simulink model "sfcndemo_matadd"  (Simulink 7.6)
settings: Solver=FixedStepDiscrete  StartTime=0.0  StopTime=10.0  RelTol=1e-3
Description:
  | Matrix-Add (Bias) Using One Input and One Parameter C-MEX S-function
settings Model: Creator=The MathWorks Inc.  ExtModeAutoUpdateStatusClock=off
settings DataIOCC: SaveOutput=off  OutputSaveName=y1,y2,y3,y4
settings OptimizationCC: BlockReduction=off  BooleanDataType=off  InlineInvariantSignals=on  InitFltsAndDblsToZero=on
settings DebuggingCC: SaveWithParameterizedLinksMsg=none  SignalResolutionControl=TryResolveAllWithWarning  SolverPrmCheckMsg=none  MultiTaskDSMMsg=warning  MultiTaskCondExecSysMsg=none
settings HardwareCC: TargetUnknown=on
settings RTWCC: IncludeERTFirstTime=on
settings CodeAppCC: CustomSymbolStrFcn=$F$N$M
settings GRTTargetCC: TargetFcnLib=ansi_tfl_tmw.mat

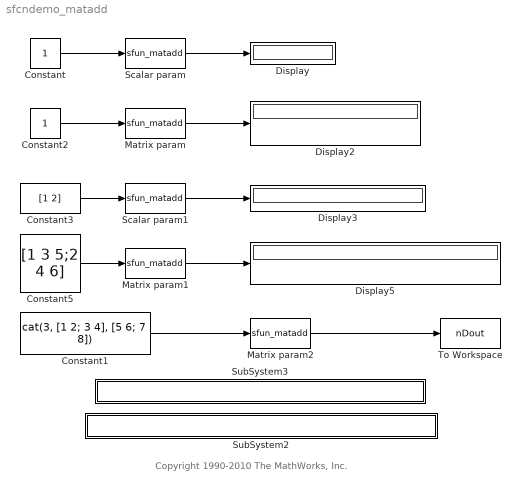
== system sfcndemo_matadd ==
  note: Copyright 1990-2010 The MathWorks, Inc.
  Constant : Constant  VectorParams1D=off
  Constant1 : Constant  Value=cat(3, [1 2; 3 4], [5 6; 7 8])  VectorParams1D=off
  Constant2 : Constant  VectorParams1D=off
  Constant3 : Constant  Value=[1 2]  VectorParams1D=off
  Constant5 : Constant  Value=[1 3 5;2 4 6]  VectorParams1D=off
  Display{,2..3,5} (4 alike) : Display
  Matrix param : S-Function  FunctionName=sfun_matadd  Parameters=Operand  EnableBusSupport=off  mask(Matrix add){Operand=[1 3; 2 4]}
      mask prompts: Operand "Operand 1:"
      settings: AttributesFormatString=Param = %<Operand>
      mask Display: disp('Matrix\n Add ')
  Matrix param1 : S-Function  FunctionName=sfun_matadd  Parameters=Operand  EnableBusSupport=off  mask(Matrix add){Operand=[1 3 5;2 4 6]}
      mask prompts: Operand "Operand 1:"
      settings: AttributesFormatString=Param = %<Operand>
      mask Display: disp('Matrix\n Add ')
  Matrix param2 : S-Function  FunctionName=sfun_matadd  Parameters=Operand  EnableBusSupport=off  mask(Matrix add){Operand=cat(3, [1 2; 3 4], [5 6; 7 8])}
      mask prompts: Operand "Operand 1:"
      settings: AttributesFormatString=Param = %<Operand>
      mask Display: disp('Matrix\n Add ')
  Scalar param : S-Function  FunctionName=sfun_matadd  Parameters=Operand  EnableBusSupport=off  mask(Matrix add){Operand=1}
      mask prompts: Operand "Operand 1:"
      settings: AttributesFormatString=Param = %<Operand>
      mask Display: disp('Matrix\n Add ')
  Scalar param1 : S-Function  FunctionName=sfun_matadd  Parameters=Operand  EnableBusSupport=off  mask(Matrix add){Operand=1}
      mask prompts: Operand "Operand 1:"
      settings: AttributesFormatString=Param = %<Operand>
      mask Display: disp('Matrix\n Add ')
  SubSystem2 : Subsystem  mask{filename=sfun_matadd.tlc}
      mask init:
      | x=sfundemo_maskdisp;
      settings: AttributesFormatString=\n  OpenFcn=sfundemo_openfcn
      mask Display: disp(x);
  SubSystem3 : Subsystem  mask{filename=sfun_matadd.c}
      mask init:
      | x=sfundemo_maskdisp;
      settings: AttributesFormatString=\n  OpenFcn=sfundemo_openfcn
      mask Display: disp(x);
  To Workspace : ToWorkspace  VariableName=nDout  SampleTime=-1  SaveFormat=Structure
  wires:
  Constant/1 -> Scalar param/1
  Scalar param/1 -> Display/1
  Constant2/1 -> Matrix param/1
  Matrix param/1 -> Display2/1
  Constant3/1 -> Scalar param1/1
  Scalar param1/1 -> Display3/1
  Constant5/1 -> Matrix param1/1
  Matrix param1/1 -> Display5/1
  Constant1/1 -> Matrix param2/1
  Matrix param2/1 -> To Workspace/1

== system sfcndemo_matadd/SubSystem2 ==

== system sfcndemo_matadd/SubSystem3 ==
